simulink model "BANSHEE_SYSTEM"  (Simulink 8.1)
settings: Solver=ode1  StartTime=0.0  StopTime=inf  FixedStep=Ts  MaxStep=1e-3  RelTol=1e-3
model workspace (MAT data in the model file):
  op_snapshot1 : opcond.OperatingPoint (value not decoded)
PostLoadFcn:
  | Ts=100e-6; BANSHEE_init;
InitFcn:
  | Ts=100e-6; BANSHEE_init;
undefined symbols (not defined in the file or in its folder): cable_spec, F1, F2, F3, Feeder1_lib, Feeder2_lib, Feeder3_lib, Left, relay_housing_lib, SM_UtilityService, SS_F1_RELAY_HOUSING, SS_F2_RELAY_HOUSING, SS_F3_RELAY_HOUSING, SS_Feeder1, SS_Feeder2, SS_Feeder3, type, utility_service_lib, V
libraries: breaker_lib x50, relay_modbus_lib x42, rtio_generic_modbus x42, cables_lib x32, artemis x24, transformer_lib x24, Load_lib x18, ssn_lib x16, rtlab x11, powerlib_extras x3, powerlib x2, LoadProfiles_lib x1
(part 1 of 3)
settings Model: ARTEMISmethode_block_infos=$$__separator__$$BANSHEE_SYSTEM/ARTEMIS Guide$$__separator__$$  Creator=RE25624  LastModifiedBy=re25624  BufferReuse=off
settings SolverCC: ZeroCrossAlgorithm=Adaptive
settings DataIOCC: ExternalInput=getinputstruct(op_snapshot1)  InitialState=getstatestruct(op_snapshot1)  LimitDataPoints=off  MaxDataPoints=90060  SignalLoggingSaveFormat=Dataset  SaveOutput=off  SignalLogging=off  DSMLogging=off  SaveTime=off  OutputSaveName=result
settings OptimizationCC: BlockReduction=off  OptimizeBlockIOStorage=off  BufferReuse=off  ExpressionFolding=off  LocalBlockOutputs=off
settings DebuggingCC: MaxConsecutiveZCsMsg=warning  IgnoredZcDiagnostic=none  SolverPrmCheckMsg=none  MultiTaskRateTransMsg=warning  FcnCallInpInsideContextMsg=EnableAllAsWarning  FrameProcessingCompatibilityMsg=error  ModelReferenceExtraNoncontSigs=warning  StrictBusMsg=None
settings ModelReferenceCC: UpdateModelReferenceTargets=IfOutOfDate
settings SFSimCC: SFSimEcho=off
settings GRTTargetCC: CodeReplacementLibrary=C89/C90 (ANSI)

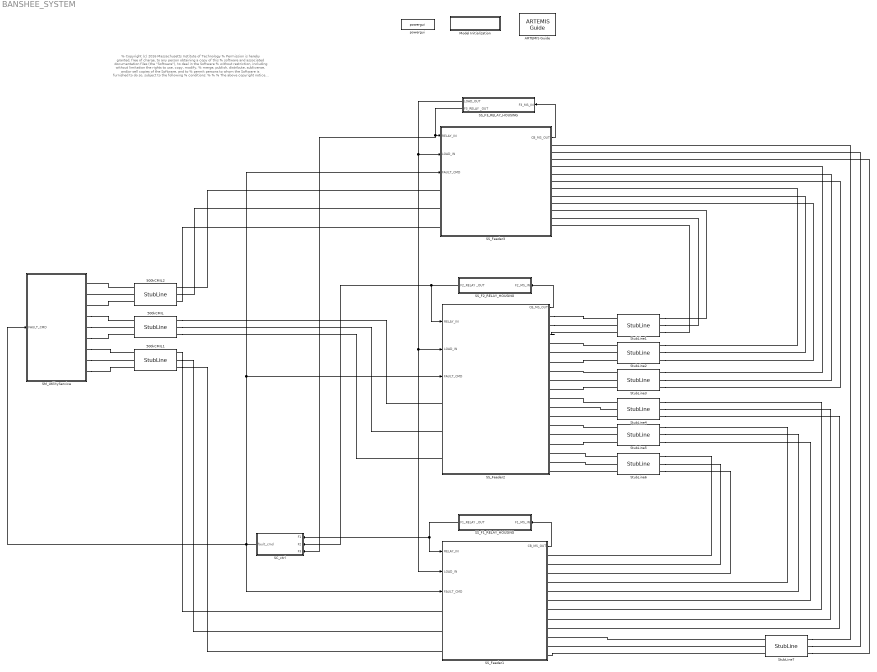
== system BANSHEE_SYSTEM ==
  note: % Copyright (c) 2016 Massachusetts Institute of Technology
      | % Permission is hereby granted, free of charge, to any person obtaining a copy of this
      | % software and associated documentation files (the "Software"), to deal in the Software
      | % without restriction, including without limitation the rights to use, copy, modify,
      | % merge, publish, distribute, sublicense, and/or sell copies of the Software, and to
      | % permit persons to whom the Software is furnished to do so, subject to the following
      | % conditions:
      | %
      | %
      | % The above copyright notice and this permission notice shall be included in
      | % all copies or substantial portions of the Software.
      | %
      | % THE SOFTWARE IS PROVIDED "AS IS", WITHOUT WARRANTY OF ANY KIND, EXPRESS OR IMPLIED,
      | % INCLUDING BUT NOT LIMITED TO THE WARRANTIES OF MERCHANTABILITY, FITNESS FOR A
      | % PARTICULAR PURPOSE AND NONINFRINGEMENT. IN NO EVENT SHALL THE AUTHORS OR COPYRIGHT
      | % HOLDERS BE LIABLE FOR ANY CLAIM, DAMAGES OR OTHER LIABILITY, WHETHER IN AN ACTION
      | % OF CONTRACT, TORT OR OTHERWISE, ARISING FROM, OUT OF OR IN CONNECTION WITH THE
      | % SOFTWARE OR THE USE OR OTHER DEALINGS IN THE SOFTWARE.
      | %
      | %
      | %%
  500kCMIL : artemis/ARTEMIS/StubLine  Phases=3  pu=off  L=10000 * 9.43453e-08 / 1  Lpu=0.08  R=10000 * 2.28409e-5 / 1  Rpu=0.002  S_base=450e6/3  V_base=230e3/sqrt(3)  F_base=60  Ts=Ts
  500kCMIL1 : artemis/ARTEMIS/StubLine  Phases=3  pu=off  L=10000 * 9.43453e-08 / 1  Lpu=0.08  R=10000 * 2.28409e-5 / 1  Rpu=0.002  S_base=450e6/3  V_base=230e3/sqrt(3)  F_base=60  Ts=Ts
  500kCMIL2 : artemis/ARTEMIS/StubLine  Phases=3  pu=off  L=10000 * 9.43453e-08 / 1  Lpu=0.08  R=10000 * 2.28409e-5 / 1  Rpu=0.002  S_base=450e6/3  V_base=230e3/sqrt(3)  F_base=60  Ts=Ts
  ARTEMIS Guide : artemis/ARTEMIS/ARTEMIS Guide  Tag=FTSSmethode_opal_4hx0r99  Description=5.0_z1  lock=on  Ts=Ts  opt=art5  dyna=off  nb_perm=4  RT_fullcomp=off  ssn=on  ssn_itvc=off  ssn_ivic=off  ssn_ext=off  ssn_solver=Art5 with Backward Euler nodal interface  ssn_impulse=off  ssn_quasimpulse=off  ssn_impulse_loop=5  paraExtinctionThy=off  Thy_Impulse=on  dtc=Off  dtc_opt=normal  ao=on  simtype=off  ct_mac=off  lin_mov=off  lsp=[0.001 2]  spike_skip=Disabled  dtc_extra=1  dtc_sws=normal  dtc_pied=0.5  SPSRulesBlock=SPSRules  tre=on  ctmm=off  LF=off  dpl_type=ARTEMiS DPL  rlc_type=off  custom_type=off  para=on  ssn_ImpulseLoopBlockedStateUpdate=5  ssn_mov_iter_number=5  ssn_switch_iter_number=5
  Model Initialization : Subsystem  AncestorBlock=artemis/Tools /Misc/Model Initialization  mask(Model Functions){InitFcnX=Ts=100e-6; BANSHEE_init;, prel=off, posl=on, inif=on, strf=off}
      mask prompts: InitFcnX "Initialisation"; prel "Preload Function"; posl "PostLoad Function"; inif "InitFcn"; strf "StartFcn"
      mask init:
      | currentBlock = gcb;
      | root = bdroot(currentBlock);
      | 
      | if ~strcmp(get_param(root,'BlockDiagramType'),'library')
      |     if prel==1
      |         set_param(root, 'PreLoadFcn', InitFcnX);
      |     else
      |         set_param(root, 'PreLoadFcn', '');
      |     end
      |     if inif==1
      |         set_param(root, 'InitFcn', InitFcnX);
      |     else
      |         set_param(root, 'InitFcn', '');
      |     end
      |     if strf==1
      |         set_param(root, 'StartFcn', InitFcnX);
      |     else
      |         set_param(root, 'StartFcn', '');
      |     end
      |     if posl==1
      |         set_param(root, 'PostLoadFcn', InitFcnX);
      |     else
      |         set_param(root, 'PostLoadFcn', '');
      |     end
      | end
      | 
      | pos = get_param(currentBlock, 'Position');
      | width = pos(3) - pos(1); height = pos(4) - pos(2);
      | txt = [ upper(root) '\n' '- InitFcn. . . . . '  get_param(root, 'InitFcn') ];
      settings: CopyFcn=set_param(gcb,'LinkStatus','inactive')
      mask Display: text(5, height*0.5, txt, 'horizontalAlignment', 'left', 'verticalAlignment', 'middle') ;
  SC_ctrl : Subsystem
  SM_UtilityService : Subsystem  AncestorBlock=utility_service_lib/SM_UtilityService
  SS_F1_RELAY_HOUSING : Subsystem  AncestorBlock=relay_housing_lib/SS_F1_RELAY_HOUSING
  SS_F2_RELAY_HOUSING : Subsystem  AncestorBlock=relay_housing_lib/SS_F2_RELAY_HOUSING
  SS_F3_RELAY_HOUSING : Subsystem  AncestorBlock=relay_housing_lib/SS_F3_RELAY_HOUSING
  SS_Feeder1 : Subsystem  AncestorBlock=Feeder1_lib/SS_Feeder1
  SS_Feeder2 : Subsystem  AncestorBlock=Feeder2_lib/SS_Feeder2
  SS_Feeder3 : Subsystem  AncestorBlock=Feeder3_lib/SS_Feeder3
  StubLine1 : artemis/ARTEMIS/StubLine  Phases=3  pu=off  L=1500 * 9.43453e-08 / 2  Lpu=0.08  R=1500 * 2.28409e-5 / 2  Rpu=0.002  S_base=450e6/3  V_base=230e3/sqrt(3)  F_base=60  Ts=Ts
  StubLine2 : artemis/ARTEMIS/StubLine  Phases=3  pu=off  L=1500 * 9.43453e-08 / 2  Lpu=0.08  R=1500 * 2.28409e-5 / 2  Rpu=0.002  S_base=450e6/3  V_base=230e3/sqrt(3)  F_base=60  Ts=Ts
  StubLine3 : artemis/ARTEMIS/StubLine  Phases=3  pu=off  L=1500 * 9.43453e-08 / 2  Lpu=0.08  R=1500 * 2.28409e-5 / 2  Rpu=0.002  S_base=450e6/3  V_base=230e3/sqrt(3)  F_base=60  Ts=Ts
  StubLine4 : artemis/ARTEMIS/StubLine  Phases=3  pu=off  L=1000 * 9.43453e-08 / 2  Lpu=0.08  R=1000 * 2.28409e-5 / 2  Rpu=0.002  S_base=450e6/3  V_base=230e3/sqrt(3)  F_base=60  Ts=Ts
  StubLine5 : artemis/ARTEMIS/StubLine  Phases=3  pu=off  L=2000 * 9.43453e-08 / 2  Lpu=0.08  R=2000 * 2.28409e-5 / 2  Rpu=0.002  S_base=450e6/3  V_base=230e3/sqrt(3)  F_base=60  Ts=Ts
  StubLine6 : artemis/ARTEMIS/StubLine  Phases=3  pu=off  L=3000 * 9.43453e-08 / 1  Lpu=0.08  R=3000 * 2.28409e-5 / 1  Rpu=0.002  S_base=450e6/3  V_base=230e3/sqrt(3)  F_base=60  Ts=Ts
  StubLine7 : artemis/ARTEMIS/StubLine  Phases=3  pu=off  L=2000 * 9.43453e-08 / 2  Lpu=0.08  R=2000 * 2.28409e-5 / 2  Rpu=0.002  S_base=450e6/3  V_base=230e3/sqrt(3)  F_base=60  Ts=Ts
  powergui : powerlib/powergui  Priority=2  SimulationMode=Discrete  SolverType=Tustin  SampleTime=Ts  frequency=60  SPID=off  DisableSnubberDevices=off  DisableRonSwitches=off  DisableVfSwitches=off  SwTol=0  Interpol=off  DisplayEquations=off  frequencyindice=0  Pbase=100e6  ErrMax=1e-4  Iterations=50  UnitsV=kV  UnitsW=MW  FunctionMessages=off  echomessages=off  HookPort=off  EnableUseOfTLC=off  x0status=blocks  RestoreLinks=warning  ResistiveCurrentMeasurement=off  Frange=logspace(0,3,50)  Ylog=off  Xlog=off  ShowGrid=off  save=off  variable=ZData  structure=0  ZoomFFT=on  StartTime=0.0  cycles=2  DisplayStyle=off  fundamental=60  FreqAxis=off  MaxFrequency=1000  frequencyindicesteady=1  RmsSteady=1  display=off  Ts=0  methode=off
  wires:
  SS_Feeder3/1(CB_MS_OUT) -> SS_F3_RELAY_HOUSING/1(F3_MS_IN)
  SS_F3_RELAY_HOUSING/2(F3_RELAY _OUT) -> SC_ctrl/3(F3), SS_Feeder3/1(RELAY_IN)
  SS_Feeder2/1(CB_MS_OUT) -> SS_F2_RELAY_HOUSING/1(F2_MS_IN)
  SS_F2_RELAY_HOUSING/1(F2_RELAY _OUT) -> SS_Feeder2/1(RELAY_IN), SC_ctrl/2(F2)
  SS_Feeder1/1(CB_MS_OUT) -> SS_F1_RELAY_HOUSING/1(F1_MS_IN)
  SS_F1_RELAY_HOUSING/1(F1_RELAY _OUT) -> SS_Feeder1/1(RELAY_IN), SC_ctrl/1(F1)
  SS_F3_RELAY_HOUSING/1(LOAD_OUT) -> SS_Feeder1/2(LOAD_IN), SS_Feeder2/2(LOAD_IN), SS_Feeder3/2(LOAD_IN)
  SC_ctrl/1(fault_cmd) -> SS_Feeder1/3(FAULT_CMD), SM_UtilityService/1(FAULT_CMD), SS_Feeder3/3(FAULT_CMD), SS_Feeder2/3(FAULT_CMD)
  connections:
  SS_Feeder2/RConn2 -- StubLine1/LConn2
  SS_Feeder2/RConn1 -- StubLine1/LConn1
  SS_Feeder2/RConn3 -- StubLine1/LConn3
  StubLine2/LConn2 -- SS_Feeder2/RConn5
  StubLine2/LConn3 -- SS_Feeder2/RConn6
  StubLine2/LConn1 -- SS_Feeder2/RConn4
  StubLine3/LConn2 -- SS_Feeder2/RConn8
  StubLine3/LConn1 -- SS_Feeder2/RConn7
  StubLine3/LConn3 -- SS_Feeder2/RConn9
  StubLine4/LConn3 -- SS_Feeder2/RConn12
  StubLine4/LConn2 -- SS_Feeder2/RConn11
  StubLine4/LConn1 -- SS_Feeder2/RConn10
  StubLine7/LConn3 -- SS_Feeder1/RConn12
  StubLine7/LConn2 -- SS_Feeder1/RConn11
  StubLine7/LConn1 -- SS_Feeder1/RConn10
  StubLine5/LConn2 -- SS_Feeder2/RConn14
  StubLine5/LConn1 -- SS_Feeder2/RConn13
  StubLine5/LConn3 -- SS_Feeder2/RConn15
  StubLine6/LConn3 -- SS_Feeder2/RConn18
  StubLine6/LConn2 -- SS_Feeder2/RConn17
  StubLine6/LConn1 -- SS_Feeder2/RConn16
  StubLine6/RConn1 -- SS_Feeder1/RConn1
  StubLine6/RConn2 -- SS_Feeder1/RConn2
  StubLine6/RConn3 -- SS_Feeder1/RConn3
  StubLine5/RConn1 -- SS_Feeder1/RConn4
  StubLine5/RConn2 -- SS_Feeder1/RConn5
  StubLine5/RConn3 -- SS_Feeder1/RConn6
  StubLine4/RConn1 -- SS_Feeder1/RConn7
  StubLine4/RConn2 -- SS_Feeder1/RConn8
  StubLine4/RConn3 -- SS_Feeder1/RConn9
  StubLine3/RConn3 -- SS_Feeder3/RConn6
  StubLine3/RConn2 -- SS_Feeder3/RConn5
  StubLine3/RConn1 -- SS_Feeder3/RConn4
  StubLine2/RConn3 -- SS_Feeder3/RConn9
  StubLine2/RConn2 -- SS_Feeder3/RConn8
  StubLine2/RConn1 -- SS_Feeder3/RConn7
  StubLine1/RConn3 -- SS_Feeder3/RConn12
  StubLine1/RConn2 -- SS_Feeder3/RConn11
  StubLine1/RConn1 -- SS_Feeder3/RConn10
  StubLine7/RConn1 -- SS_Feeder3/RConn1
  StubLine7/RConn2 -- SS_Feeder3/RConn2
  StubLine7/RConn3 -- SS_Feeder3/RConn3
  500kCMIL2/LConn2 -- SM_UtilityService/RConn2
  500kCMIL2/LConn1 -- SM_UtilityService/RConn1
  500kCMIL2/LConn3 -- SM_UtilityService/RConn3
  SM_UtilityService/RConn5 -- 500kCMIL/LConn2
  SM_UtilityService/RConn6 -- 500kCMIL/LConn3
  SM_UtilityService/RConn4 -- 500kCMIL/LConn1
  SM_UtilityService/RConn8 -- 500kCMIL1/LConn2
  SM_UtilityService/RConn7 -- 500kCMIL1/LConn1
  SM_UtilityService/RConn9 -- 500kCMIL1/LConn3
  500kCMIL2/RConn3 -- SS_Feeder3/LConn3
  500kCMIL2/RConn2 -- SS_Feeder3/LConn2
  500kCMIL2/RConn1 -- SS_Feeder3/LConn1
  500kCMIL/RConn1 -- SS_Feeder2/LConn1
  500kCMIL/RConn2 -- SS_Feeder2/LConn2
  500kCMIL/RConn3 -- SS_Feeder2/LConn3
  500kCMIL1/RConn1 -- SS_Feeder1/LConn1
  500kCMIL1/RConn2 -- SS_Feeder1/LConn2
  500kCMIL1/RConn3 -- SS_Feeder1/LConn3

== system BANSHEE_SYSTEM/Model Initialization ==

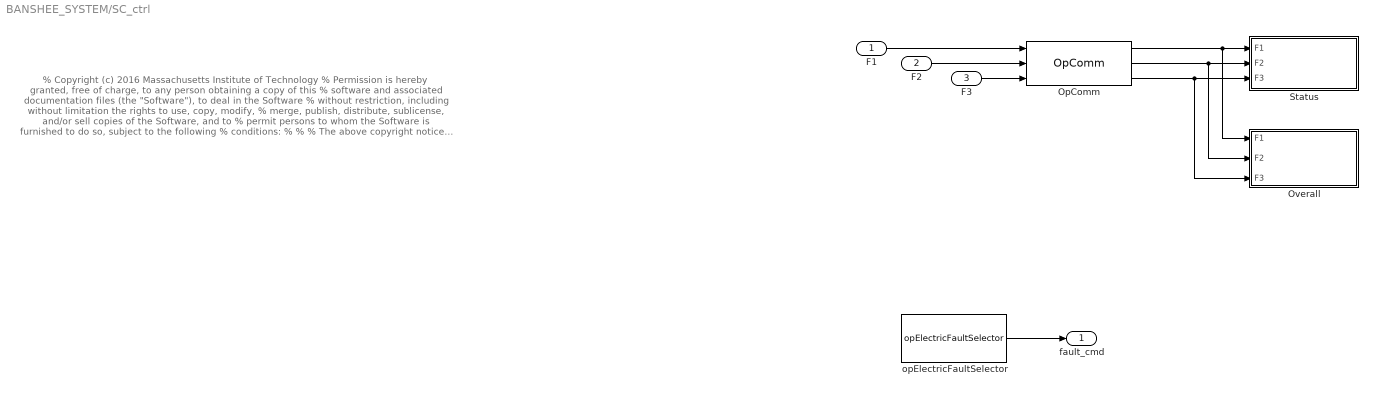
== system BANSHEE_SYSTEM/SC_ctrl ==
  note: % Copyright (c) 2016 Massachusetts Institute of Technology
      | % Permission is hereby granted, free of charge, to any person obtaining a copy of this
      | % software and associated documentation files (the "Software"), to deal in the Software
      | % without restriction, including without limitation the rights to use, copy, modify,
      | % merge, publish, distribute, sublicense, and/or sell copies of the Software, and to
      | % permit persons to whom the Software is furnished to do so, subject to the following
      | % conditions:
      | %
      | %
      | % The above copyright notice and this permission notice shall be included in
      | % all copies or substantial portions of the Software.
      | %
      | % THE SOFTWARE IS PROVIDED "AS IS", WITHOUT WARRANTY OF ANY KIND, EXPRESS OR IMPLIED,
      | % INCLUDING BUT NOT LIMITED TO THE WARRANTIES OF MERCHANTABILITY, FITNESS FOR A
      | % PARTICULAR PURPOSE AND NONINFRINGEMENT. IN NO EVENT SHALL THE AUTHORS OR COPYRIGHT
      | % HOLDERS BE LIABLE FOR ANY CLAIM, DAMAGES OR OTHER LIABILITY, WHETHER IN AN ACTION
      | % OF CONTRACT, TORT OR OTHERWISE, ARISING FROM, OUT OF OR IN CONNECTION WITH THE
      | % SOFTWARE OR THE USE OR OTHER DEALINGS IN THE SOFTWARE.
      | %
      | %
      | %%
  F1 : Inport
  F2 : Inport  Port=2
  F3 : Inport  Port=3
  OpComm : rtlab/OpComm  nbport=3  groupe_acq=1  subsys_rate=0  st=0  Synchronization=on  Interpolation=on  Threshold=1.0  Missed_Data=off  Sim_Time=off  Samples=off  dynSigOut=off  from_console=0  warning_done=off  writeOpCommFile=off  Offset=off
  Overall : Subsystem
  Status : Subsystem
  opElectricFaultSelector : artemis/Tools /POW faults/opElectricFaultSelector  phase_a=on  phase_b=on  phase_c=on  gnd_fault=on  Tacq=1  Tst=[0.1 0 10]  enable_POW=off  angle_POW=[15 0 10]  Tdr="[0.5 0  10]"  fault_location_menu=No fault  T_init=2
  fault_cmd : Outport
  wires:
  F1/1 -> OpComm/1
  F2/1 -> OpComm/2
  F3/1 -> OpComm/3
  OpComm/1 -> Overall/1(F1), Status/1(F1)
  OpComm/2 -> Overall/2(F2), Status/2(F2)
  OpComm/3 -> Overall/3(F3), Status/3(F3)
  opElectricFaultSelector/1 -> fault_cmd/1

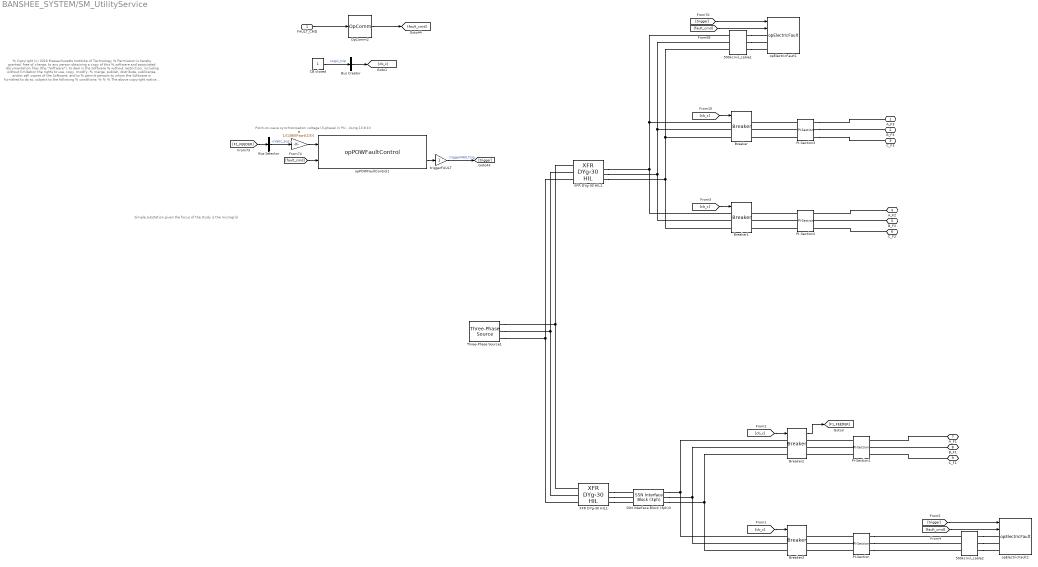
== system BANSHEE_SYSTEM/SM_UtilityService ==
  note: Simple substation given the focus of the study is the microgrid
  note: % Copyright (c) 2016 Massachusetts Institute of Technology
      | % Permission is hereby granted, free of charge, to any person obtaining a copy of this
      | % software and associated documentation files (the "Software"), to deal in the Software
      | % without restriction, including without limitation the rights to use, copy, modify,
      | % merge, publish, distribute, sublicense, and/or sell copies of the Software, and to
      | % permit persons to whom the Software is furnished to do so, subject to the following
      | % conditions:
      | %
      | %
      | % The above copyright notice and this permission notice shall be included in
      | % all copies or substantial portions of the Software.
      | %
      | % THE SOFTWARE IS PROVIDED "AS IS", WITHOUT WARRANTY OF ANY KIND, EXPRESS OR IMPLIED,
      | % INCLUDING BUT NOT LIMITED TO THE WARRANTIES OF MERCHANTABILITY, FITNESS FOR A
      | % PARTICULAR PURPOSE AND NONINFRINGEMENT. IN NO EVENT SHALL THE AUTHORS OR COPYRIGHT
      | % HOLDERS BE LIABLE FOR ANY CLAIM, DAMAGES OR OTHER LIABILITY, WHETHER IN AN ACTION
      | % OF CONTRACT, TORT OR OTHERWISE, ARISING FROM, OUT OF OR IN CONNECTION WITH THE
      | % SOFTWARE OR THE USE OR OTHER DEALINGS IN THE SOFTWARE.
      | %
      | %
      | %%
  note: Point-on-wave synchronisation voltage (3-phase) in PU - Using 13.8 kV
  FAULT_CMD : Inport
  500kcmil_cable1 : cables_lib/500kcmil_cable  length=1  par_sets=1
  500kcmil_cable2 : cables_lib/500kcmil_cable  length=1  par_sets=1
  Breaker{,1..3} (4 alike) : breaker_lib/Breaker  Ts=Ts
  Bus Creator : BusCreator  Inputs=1
  Bus Selector : BusSelector  OutputSignals=Vabc_bus
  CB closed : Constant
  OpComm2 : rtlab/OpComm  nbport=1  groupe_acq=1  subsys_rate=0  st=0  Synchronization=on  Interpolation=on  Threshold=1.0  Missed_Data=off  Sim_Time=off  Samples=off  dynSigOut=off  from_console=1  warning_done=off  writeOpCommFile=off  Offset=off
  PI-Section : cables_lib/PI-Section  cable_spec=[cable_spec(13, :)]  line_length=3000  parallel_sets=1
  PI-Section1 : cables_lib/PI-Section  cable_spec=[cable_spec(13, :)]  line_length=500  parallel_sets=1
  PI-Section2 : cables_lib/PI-Section  cable_spec=[cable_spec(13, :)]  line_length=500  parallel_sets=1
  PI-Section3 : cables_lib/PI-Section  cable_spec=[cable_spec(13, :)]  line_length=500  parallel_sets=1
  SSN Interface Block (3ph)3 : ssn_lib/SSN Interface Block (3ph)  nb_phase=3  nb_port=2  p1_type=V-type(Left)  p2_type=V-type (Right)  p3_type=V-type(Left)  p4_type=V-type(Left)  p5_type=V-type(Left)  p6_type=V-type(Left)  p7_type=V-type(Left)  p8_type=V-type(Left)  p9_type=V-type(Left)  p10_type=V-type(Left)  p11_type=V-type(Left)  p12_type=V-type(Left)  p13_type=V-type(Left)  p14_type=V-type(Left)  p15_type=V-type(Left)  p16_type=V-type(Left)  I_port_shunt_resistance=1e9
  Three-Phase Source1 : powerlib/Electrical Sources/Three-Phase Source  Voltage=115000  PhaseAngle=0  Frequency=60  InternalConnection=Yg  SpecifyImpedance=on  Resistance=0.8929  Inductance=16.58e-3  ShortCircuitLevel=100e6  BaseVoltage=115000  XRratio=30  BusType=swing  Pref=0  Qref=0  Qmin=-inf  Qmax=inf
  XFR DYg-30 HIL1 : transformer_lib/XFR DYg-30 HIL  Rating=50000  Vp=115000  Vs=13800  Z=15  XR=30
  XFR DYg-30 HIL2 : transformer_lib/XFR DYg-30 HIL  Rating=50000  Vp=115000  Vs=13800  Z=15  XR=30
  a : Gain  Gain=1/(13800*sqrt(2/3))
  opElectricFault1 : artemis/Tools /POW faults/opElectricFault  FaultLocation=location 7  FaultResistance=0.0001  GroundResistance=0.0001  InitialStates=[0 0 0]  SnubberResistance=1e6  SnubberCapacitance=inf
  opElectricFault2 : artemis/Tools /POW faults/opElectricFault  FaultLocation=location 8  FaultResistance=0.0001  GroundResistance=0.0001  InitialStates=[0 0 0]  SnubberResistance=1e6  SnubberCapacitance=inf
  opPOWFaultControl1 : artemis/Tools /POW faults/opPOWFaultControl  Ts=Ts  usePLL=off  Fgrid=60  PLL_k=[180 3200 1]  vol_sel=1: rising zero-corssing  SyncPhase_menu=A  T_acq=0.8
  triggerFAULT : Gain
  A_F3 : PMIOPort  Port=1  Side=Right
  B_F3 : PMIOPort  Port=2  Side=Right
  C_F3 : PMIOPort  Port=3  Side=Right
  A_F2 : PMIOPort  Port=4  Side=Right
  B_F2 : PMIOPort  Port=5  Side=Right
  C_F2 : PMIOPort  Port=6  Side=Right
  A_F1 : PMIOPort  Port=7  Side=Right
  B_F1 : PMIOPort  Port=8  Side=Right
  C_F1 : PMIOPort  Port=9  Side=Right
  wires:
  [cb_c] -> Breaker2/1
  [cb_c] -> Breaker/1
  [cb_c] -> Breaker1/1
  [cb_c] -> Breaker3/1
  Bus Creator/1 -> [cb_c]
  CB closed/1 -> Bus Creator/1  "Logic_trip"
  [fault_cmd] -> opElectricFault1/2
  [trigger] -> opElectricFault1/1
  [fault_cmd] -> opPOWFaultControl1/2
  opPOWFaultControl1/2 -> triggerFAULT/1
  triggerFAULT/1 -> [trigger]  "triggerFAULTsig"
  [F1_FEEDER] -> Bus Selector/1
  Bus Selector/1 -> a/1  "<Vabc_bus>"
  a/1 -> opPOWFaultControl1/1
  OpComm2/1 -> [fault_cmd]
  FAULT_CMD/1 -> OpComm2/1
  Breaker2/1 -> [F1_FEEDER]
  [fault_cmd] -> opElectricFault2/2
  [trigger] -> opElectricFault2/1
  connections:
  PI-Section2/LConn1 -- Breaker1/RConn1
  PI-Section2/LConn3 -- Breaker1/RConn3
  PI-Section1/LConn1 -- Breaker2/RConn1
  PI-Section1/LConn2 -- Breaker2/RConn2
  PI-Section3/LConn1 -- Breaker/RConn1
  PI-Section1/LConn3 -- Breaker2/RConn3
  Breaker3/LConn2 -- SSN Interface Block (3ph)3/RConn2 -- Breaker2/LConn2
  PI-Section3/LConn2 -- Breaker/RConn2
  Breaker3/LConn3 -- SSN Interface Block (3ph)3/RConn3 -- Breaker2/LConn3
  PI-Section/LConn3 -- Breaker3/RConn3
  PI-Section2/LConn2 -- Breaker1/RConn2
  PI-Section/LConn1 -- Breaker3/RConn1
  Breaker3/LConn1 -- SSN Interface Block (3ph)3/RConn1 -- Breaker2/LConn1
  PI-Section3/LConn3 -- Breaker/RConn3
  Breaker1/LConn2 -- 500kcmil_cable1/LConn2 -- Breaker/LConn2 -- XFR DYg-30 HIL2/RConn2
  XFR DYg-30 HIL2/RConn1 -- Breaker1/LConn1 -- 500kcmil_cable1/LConn1 -- Breaker/LConn1
  Breaker1/LConn3 -- 500kcmil_cable1/LConn3 -- Breaker/LConn3 -- XFR DYg-30 HIL2/RConn3
  PI-Section/LConn2 -- Breaker3/RConn2
  A_F2/RConn1 -- PI-Section2/RConn1
  B_F1/RConn1 -- PI-Section1/RConn2
  PI-Section3/RConn3 -- C_F3/RConn1
  Three-Phase Source1/RConn3 -- XFR DYg-30 HIL2/LConn3 -- XFR DYg-30 HIL1/LConn3
  Three-Phase Source1/RConn2 -- XFR DYg-30 HIL2/LConn2 -- XFR DYg-30 HIL1/LConn2
  Three-Phase Source1/RConn1 -- XFR DYg-30 HIL2/LConn1 -- XFR DYg-30 HIL1/LConn1
  C_F2/RConn1 -- PI-Section2/RConn3
  PI-Section3/RConn1 -- A_F3/RConn1
  B_F2/RConn1 -- PI-Section2/RConn2
  A_F1/RConn1 -- PI-Section1/RConn1
  C_F1/RConn1 -- PI-Section1/RConn3
  PI-Section3/RConn2 -- B_F3/RConn1
  500kcmil_cable1/RConn3 -- opElectricFault1/LConn3
  500kcmil_cable1/RConn2 -- opElectricFault1/LConn2
  500kcmil_cable1/RConn1 -- opElectricFault1/LConn1
  500kcmil_cable2/RConn3 -- opElectricFault2/LConn3
  500kcmil_cable2/RConn2 -- opElectricFault2/LConn2
  500kcmil_cable2/RConn1 -- opElectricFault2/LConn1
  PI-Section/RConn3 -- 500kcmil_cable2/LConn3
  PI-Section/RConn2 -- 500kcmil_cable2/LConn2
  PI-Section/RConn1 -- 500kcmil_cable2/LConn1
  XFR DYg-30 HIL1/RConn3 -- SSN Interface Block (3ph)3/LConn3
  XFR DYg-30 HIL1/RConn2 -- SSN Interface Block (3ph)3/LConn2
  XFR DYg-30 HIL1/RConn1 -- SSN Interface Block (3ph)3/LConn1

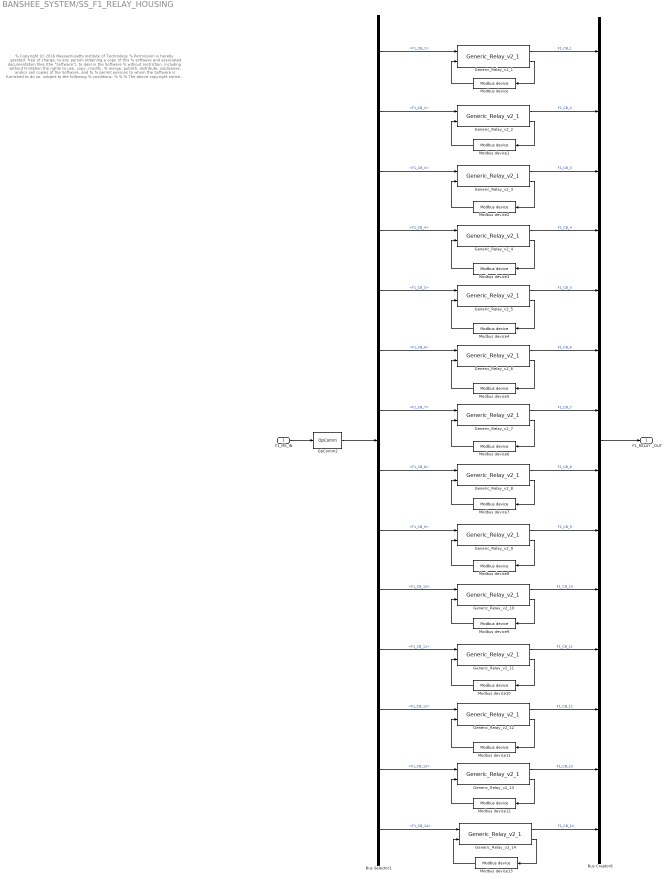
== system BANSHEE_SYSTEM/SS_F1_RELAY_HOUSING ==
  note: % Copyright (c) 2016 Massachusetts Institute of Technology
      | % Permission is hereby granted, free of charge, to any person obtaining a copy of this
      | % software and associated documentation files (the "Software"), to deal in the Software
      | % without restriction, including without limitation the rights to use, copy, modify,
      | % merge, publish, distribute, sublicense, and/or sell copies of the Software, and to
      | % permit persons to whom the Software is furnished to do so, subject to the following
      | % conditions:
      | %
      | %
      | % The above copyright notice and this permission notice shall be included in
      | % all copies or substantial portions of the Software.
      | %
      | % THE SOFTWARE IS PROVIDED "AS IS", WITHOUT WARRANTY OF ANY KIND, EXPRESS OR IMPLIED,
      | % INCLUDING BUT NOT LIMITED TO THE WARRANTIES OF MERCHANTABILITY, FITNESS FOR A
      | % PARTICULAR PURPOSE AND NONINFRINGEMENT. IN NO EVENT SHALL THE AUTHORS OR COPYRIGHT
      | % HOLDERS BE LIABLE FOR ANY CLAIM, DAMAGES OR OTHER LIABILITY, WHETHER IN AN ACTION
      | % OF CONTRACT, TORT OR OTHERWISE, ARISING FROM, OUT OF OR IN CONNECTION WITH THE
      | % SOFTWARE OR THE USE OR OTHER DEALINGS IN THE SOFTWARE.
      | %
      | %
      | %%
  F1_MS_IN : Inport
  Bus Creator6 : BusCreator  Inputs=14
  Bus Selector1 : BusSelector  OutputSignals=F1_CB_1,F1_CB_2,F1_CB_3,F1_CB_4,F1_CB_5,F1_CB_6,F1_CB_7,F1_CB_8,F1_CB_9,F1_CB_10,F1_CB_11,F1_CB_12,F1_CB_13,F1_CB_14
  Generic_Relay_v2_1 : relay_modbus_lib/Generic_Relay_v2_1  Ts=Ts  relay_settings=[F1(1,:)]
  Generic_Relay_v2_10 : relay_modbus_lib/Generic_Relay_v2_1  Ts=Ts  relay_settings=[F1(10,:)]
  Generic_Relay_v2_11 : relay_modbus_lib/Generic_Relay_v2_1  Ts=Ts  relay_settings=[F1(11,:)]
  Generic_Relay_v2_12 : relay_modbus_lib/Generic_Relay_v2_1  Ts=Ts  relay_settings=[F1(12,:)]
  Generic_Relay_v2_13 : relay_modbus_lib/Generic_Relay_v2_1  Ts=Ts  relay_settings=[F1(13,:)]
  Generic_Relay_v2_14 : relay_modbus_lib/Generic_Relay_v2_1  Ts=Ts  relay_settings=[F1(14,:)]
  Generic_Relay_v2_2 : relay_modbus_lib/Generic_Relay_v2_1  Ts=Ts  relay_settings=[F1(2,:)]
  Generic_Relay_v2_3 : relay_modbus_lib/Generic_Relay_v2_1  Ts=Ts  relay_settings=[F1(3,:)]
  Generic_Relay_v2_4 : relay_modbus_lib/Generic_Relay_v2_1  Ts=Ts  relay_settings=[F1(4,:)]
  Generic_Relay_v2_5 : relay_modbus_lib/Generic_Relay_v2_1  Ts=Ts  relay_settings=[F1(5,:)]
  Generic_Relay_v2_6 : relay_modbus_lib/Generic_Relay_v2_1  Ts=Ts  relay_settings=[F1(6,:)]
  Generic_Relay_v2_7 : relay_modbus_lib/Generic_Relay_v2_1  Ts=Ts  relay_settings=[F1(7,:)]
  Generic_Relay_v2_8 : relay_modbus_lib/Generic_Relay_v2_1  Ts=Ts  relay_settings=[F1(8,:)]
  Generic_Relay_v2_9 : relay_modbus_lib/Generic_Relay_v2_1  Ts=Ts  relay_settings=[F1(9,:)]
  Modbus device : rtio_generic_modbus/Modbus device  conf_name=F1_relay_cfg1.opal  conf_name_mask=F1_relay_cfg1.xls  sample_time=Ts
  Modbus device1 : rtio_generic_modbus/Modbus device  conf_name=F1_relay_cfg2.opal  conf_name_mask=F1_relay_cfg2.xls  sample_time=Ts
  Modbus device10 : rtio_generic_modbus/Modbus device  conf_name=F1_relay_cfg11.opal  conf_name_mask=F1_relay_cfg11.xls  sample_time=Ts
  Modbus device11 : rtio_generic_modbus/Modbus device  conf_name=F1_relay_cfg12.opal  conf_name_mask=F1_relay_cfg12.xls  sample_time=Ts
  Modbus device12 : rtio_generic_modbus/Modbus device  conf_name=F1_relay_cfg13.opal  conf_name_mask=F1_relay_cfg13.xls  sample_time=Ts
  Modbus device13 : rtio_generic_modbus/Modbus device  conf_name=F1_relay_cfg14.opal  conf_name_mask=F1_relay_cfg14.xls  sample_time=Ts
  Modbus device2 : rtio_generic_modbus/Modbus device  conf_name=F1_relay_cfg3.opal  conf_name_mask=F1_relay_cfg3.xls  sample_time=Ts
  Modbus device3 : rtio_generic_modbus/Modbus device  conf_name=F1_relay_cfg4.opal  conf_name_mask=F1_relay_cfg4.xls  sample_time=Ts
  Modbus device4 : rtio_generic_modbus/Modbus device  conf_name=F1_relay_cfg5.opal  conf_name_mask=F1_relay_cfg5.xls  sample_time=Ts
  Modbus device5 : rtio_generic_modbus/Modbus device  conf_name=F1_relay_cfg6.opal  conf_name_mask=F1_relay_cfg6.xls  sample_time=Ts
  Modbus device6 : rtio_generic_modbus/Modbus device  conf_name=F1_relay_cfg7.opal  conf_name_mask=F1_relay_cfg7.xls  sample_time=Ts
  Modbus device7 : rtio_generic_modbus/Modbus device  conf_name=F1_relay_cfg8.opal  conf_name_mask=F1_relay_cfg8.xls  sample_time=Ts
  Modbus device8 : rtio_generic_modbus/Modbus device  conf_name=F1_relay_cfg9.opal  conf_name_mask=F1_relay_cfg9.xls  sample_time=Ts
  Modbus device9 : rtio_generic_modbus/Modbus device  conf_name=F1_relay_cfg10.opal  conf_name_mask=F1_relay_cfg10.xls  sample_time=Ts
  OpComm2 : rtlab/OpComm  nbport=1  groupe_acq=1  subsys_rate=0  st=0  Synchronization=on  Interpolation=on  Threshold=1.0  Missed_Data=off  Sim_Time=off  Samples=off  dynSigOut=off  from_console=0  warning_done=off  writeOpCommFile=off  Offset=off
  F1_RELAY _OUT : Outport
  wires:
  OpComm2/1 -> Bus Selector1/1
  Modbus device12/1 -> Generic_Relay_v2_13/2
  Generic_Relay_v2_13/2 -> Modbus device12/1
  Modbus device11/1 -> Generic_Relay_v2_12/2
  Generic_Relay_v2_12/2 -> Modbus device11/1
  Modbus device10/1 -> Generic_Relay_v2_11/2
  Generic_Relay_v2_11/2 -> Modbus device10/1
  Modbus device9/1 -> Generic_Relay_v2_10/2
  Generic_Relay_v2_10/2 -> Modbus device9/1
  Modbus device8/1 -> Generic_Relay_v2_9/2
  Generic_Relay_v2_9/2 -> Modbus device8/1
  Modbus device7/1 -> Generic_Relay_v2_8/2
  Generic_Relay_v2_8/2 -> Modbus device7/1
  Modbus device6/1 -> Generic_Relay_v2_7/2
  Generic_Relay_v2_7/2 -> Modbus device6/1
  Modbus device5/1 -> Generic_Relay_v2_6/2
  Generic_Relay_v2_6/2 -> Modbus device5/1
  Modbus device4/1 -> Generic_Relay_v2_5/2
  Generic_Relay_v2_5/2 -> Modbus device4/1
  Modbus device3/1 -> Generic_Relay_v2_4/2
  Generic_Relay_v2_4/2 -> Modbus device3/1
  Modbus device2/1 -> Generic_Relay_v2_3/2
  Generic_Relay_v2_3/2 -> Modbus device2/1
  Generic_Relay_v2_2/2 -> Modbus device1/1
  Modbus device1/1 -> Generic_Relay_v2_2/2
  Generic_Relay_v2_1/2 -> Modbus device/1
  Modbus device/1 -> Generic_Relay_v2_1/2
  F1_MS_IN/1 -> OpComm2/1
  Bus Selector1/1 -> Generic_Relay_v2_1/1  "<F1_CB_1>"
  Generic_Relay_v2_1/1 -> Bus Creator6/1  "F1_CB_1"
  Bus Creator6/1 -> F1_RELAY _OUT/1
  Bus Selector1/2 -> Generic_Relay_v2_2/1  "<F1_CB_2>"
  Generic_Relay_v2_2/1 -> Bus Creator6/2  "F1_CB_2"
  Bus Selector1/3 -> Generic_Relay_v2_3/1  "<F1_CB_3>"
  Bus Selector1/4 -> Generic_Relay_v2_4/1  "<F1_CB_4>"
  Bus Selector1/5 -> Generic_Relay_v2_5/1  "<F1_CB_5>"
  Bus Selector1/6 -> Generic_Relay_v2_6/1  "<F1_CB_6>"
  Bus Selector1/7 -> Generic_Relay_v2_7/1  "<F1_CB_7>"
  Bus Selector1/8 -> Generic_Relay_v2_8/1  "<F1_CB_8>"
  Bus Selector1/9 -> Generic_Relay_v2_9/1  "<F1_CB_9>"
  Bus Selector1/10 -> Generic_Relay_v2_10/1  "<F1_CB_10>"
  Bus Selector1/11 -> Generic_Relay_v2_11/1  "<F1_CB_11>"
  Bus Selector1/12 -> Generic_Relay_v2_12/1  "<F1_CB_12>"
  Bus Selector1/13 -> Generic_Relay_v2_13/1  "<F1_CB_13>"
  Generic_Relay_v2_13/1 -> Bus Creator6/13  "F1_CB_13"
  Generic_Relay_v2_12/1 -> Bus Creator6/12  "F1_CB_12"
  Generic_Relay_v2_11/1 -> Bus Creator6/11  "F1_CB_11"
  Generic_Relay_v2_10/1 -> Bus Creator6/10  "F1_CB_10"
  Generic_Relay_v2_9/1 -> Bus Creator6/9  "F1_CB_9"
  Generic_Relay_v2_8/1 -> Bus Creator6/8  "F1_CB_8"
  Generic_Relay_v2_7/1 -> Bus Creator6/7  "F1_CB_7"
  Generic_Relay_v2_6/1 -> Bus Creator6/6  "F1_CB_6"
  Generic_Relay_v2_5/1 -> Bus Creator6/5  "F1_CB_5"
  Generic_Relay_v2_4/1 -> Bus Creator6/4  "F1_CB_4"
  Generic_Relay_v2_3/1 -> Bus Creator6/3  "F1_CB_3"
  Modbus device13/1 -> Generic_Relay_v2_14/2
  Generic_Relay_v2_14/2 -> Modbus device13/1
  Generic_Relay_v2_14/1 -> Bus Creator6/14  "F1_CB_14"
  Bus Selector1/14 -> Generic_Relay_v2_14/1  "<F1_CB_14>"

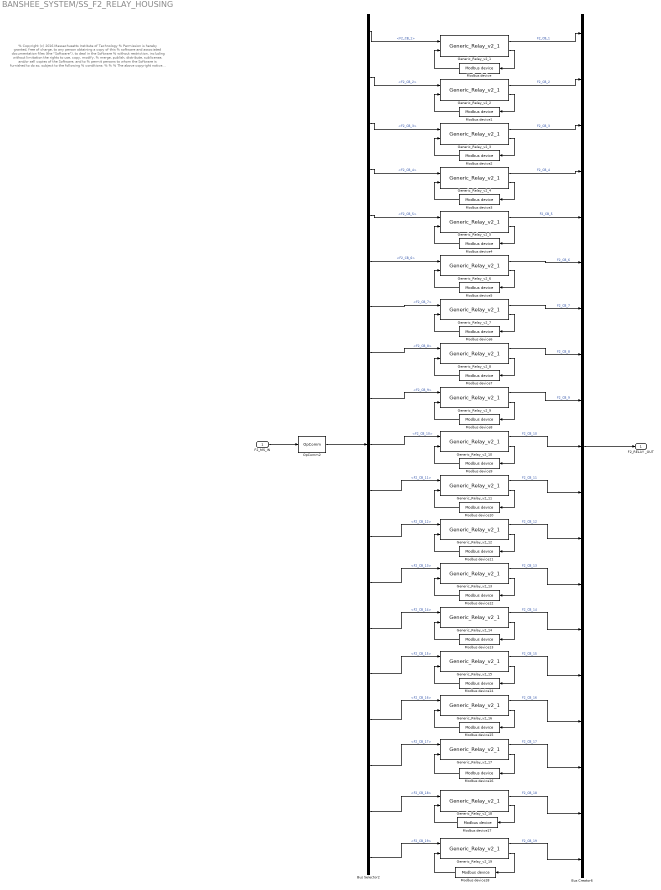
== system BANSHEE_SYSTEM/SS_F2_RELAY_HOUSING ==
  note: % Copyright (c) 2016 Massachusetts Institute of Technology
      | % Permission is hereby granted, free of charge, to any person obtaining a copy of this
      | % software and associated documentation files (the "Software"), to deal in the Software
      | % without restriction, including without limitation the rights to use, copy, modify,
      | % merge, publish, distribute, sublicense, and/or sell copies of the Software, and to
      | % permit persons to whom the Software is furnished to do so, subject to the following
      | % conditions:
      | %
      | %
      | % The above copyright notice and this permission notice shall be included in
      | % all copies or substantial portions of the Software.
      | %
      | % THE SOFTWARE IS PROVIDED "AS IS", WITHOUT WARRANTY OF ANY KIND, EXPRESS OR IMPLIED,
      | % INCLUDING BUT NOT LIMITED TO THE WARRANTIES OF MERCHANTABILITY, FITNESS FOR A
      | % PARTICULAR PURPOSE AND NONINFRINGEMENT. IN NO EVENT SHALL THE AUTHORS OR COPYRIGHT
      | % HOLDERS BE LIABLE FOR ANY CLAIM, DAMAGES OR OTHER LIABILITY, WHETHER IN AN ACTION
      | % OF CONTRACT, TORT OR OTHERWISE, ARISING FROM, OUT OF OR IN CONNECTION WITH THE
      | % SOFTWARE OR THE USE OR OTHER DEALINGS IN THE SOFTWARE.
      | %
      | %
      | %%
  F2_MS_IN : Inport
  Bus Creator6 : BusCreator  Inputs=19
  Bus Selector2 : BusSelector  OutputSignals=F2_CB_1,F2_CB_2,F2_CB_3,F2_CB_4,F2_CB_5,F2_CB_6,F2_CB_7,F2_CB_8,F2_CB_9,F2_CB_10,F2_CB_11,F2_CB_12,F2_CB_13,F2_CB_14,F2_CB_15,F2_CB_16,F2_CB_17,F2_CB_18,F2_CB_19
  Generic_Relay_v2_1 : relay_modbus_lib/Generic_Relay_v2_1  Ts=Ts  relay_settings=[F2(1,:)]
  Generic_Relay_v2_10 : relay_modbus_lib/Generic_Relay_v2_1  Ts=Ts  relay_settings=[F2(10,:)]
  Generic_Relay_v2_11 : relay_modbus_lib/Generic_Relay_v2_1  Ts=Ts  relay_settings=[F2(11,:)]
  Generic_Relay_v2_12 : relay_modbus_lib/Generic_Relay_v2_1  Ts=Ts  relay_settings=[F2(12,:)]
  Generic_Relay_v2_13 : relay_modbus_lib/Generic_Relay_v2_1  Ts=Ts  relay_settings=[F2(13,:)]
  Generic_Relay_v2_14 : relay_modbus_lib/Generic_Relay_v2_1  Ts=Ts  relay_settings=[F2(14,:)]
  Generic_Relay_v2_15 : relay_modbus_lib/Generic_Relay_v2_1  Ts=Ts  relay_settings=[F2(15,:)]
  Generic_Relay_v2_16 : relay_modbus_lib/Generic_Relay_v2_1  Ts=Ts  relay_settings=[F2(16,:)]
  Generic_Relay_v2_17 : relay_modbus_lib/Generic_Relay_v2_1  Ts=Ts  relay_settings=[F2(17,:)]
  Generic_Relay_v2_18 : relay_modbus_lib/Generic_Relay_v2_1  Ts=Ts  relay_settings=[F2(18,:)]
  Generic_Relay_v2_19 : relay_modbus_lib/Generic_Relay_v2_1  Ts=Ts  relay_settings=[F2(19,:)]
  Generic_Relay_v2_2 : relay_modbus_lib/Generic_Relay_v2_1  Ts=Ts  relay_settings=[F2(2,:)]
  Generic_Relay_v2_3 : relay_modbus_lib/Generic_Relay_v2_1  Ts=Ts  relay_settings=[F2(3,:)]
  Generic_Relay_v2_4 : relay_modbus_lib/Generic_Relay_v2_1  Ts=Ts  relay_settings=[F2(4,:)]
  Generic_Relay_v2_5 : relay_modbus_lib/Generic_Relay_v2_1  Ts=Ts  relay_settings=[F2(5,:)]
  Generic_Relay_v2_6 : relay_modbus_lib/Generic_Relay_v2_1  Ts=Ts  relay_settings=[F2(6,:)]
  Generic_Relay_v2_7 : relay_modbus_lib/Generic_Relay_v2_1  Ts=Ts  relay_settings=[F2(7,:)]
  Generic_Relay_v2_8 : relay_modbus_lib/Generic_Relay_v2_1  Ts=Ts  relay_settings=[F2(8,:)]
  Generic_Relay_v2_9 : relay_modbus_lib/Generic_Relay_v2_1  Ts=Ts  relay_settings=[F2(9,:)]
  Modbus device : rtio_generic_modbus/Modbus device  conf_name=F2_relay_cfg1.opal  conf_name_mask=F2_relay_cfg1.xls  sample_time=Ts
  Modbus device1 : rtio_generic_modbus/Modbus device  conf_name=F2_relay_cfg2.opal  conf_name_mask=F2_relay_cfg2.xls  sample_time=Ts
  Modbus device10 : rtio_generic_modbus/Modbus device  conf_name=F2_relay_cfg11.opal  conf_name_mask=F2_relay_cfg11.xls  sample_time=Ts
  Modbus device11 : rtio_generic_modbus/Modbus device  conf_name=F2_relay_cfg12.opal  conf_name_mask=F2_relay_cfg12.xls  sample_time=Ts
  Modbus device12 : rtio_generic_modbus/Modbus device  conf_name=F2_relay_cfg13.opal  conf_name_mask=F2_relay_cfg13.xls  sample_time=Ts
  Modbus device13 : rtio_generic_modbus/Modbus device  conf_name=F2_relay_cfg14.opal  conf_name_mask=F2_relay_cfg14.xls  sample_time=Ts
  Modbus device14 : rtio_generic_modbus/Modbus device  conf_name=F2_relay_cfg15.opal  conf_name_mask=F2_relay_cfg15.xls  sample_time=Ts
  Modbus device15 : rtio_generic_modbus/Modbus device  conf_name=F2_relay_cfg16.opal  conf_name_mask=F2_relay_cfg16.xls  sample_time=Ts
  Modbus device16 : rtio_generic_modbus/Modbus device  conf_name=F2_relay_cfg17.opal  conf_name_mask=F2_relay_cfg17.xls  sample_time=Ts
  Modbus device17 : rtio_generic_modbus/Modbus device  conf_name=F2_relay_cfg18.opal  conf_name_mask=F2_relay_cfg18.xls  sample_time=Ts
  Modbus device18 : rtio_generic_modbus/Modbus device  conf_name=F2_relay_cfg19.opal  conf_name_mask=F2_relay_cfg19.xls  sample_time=Ts
  Modbus device2 : rtio_generic_modbus/Modbus device  conf_name=F2_relay_cfg3.opal  conf_name_mask=F2_relay_cfg3.xls  sample_time=Ts
  Modbus device3 : rtio_generic_modbus/Modbus device  conf_name=F2_relay_cfg4.opal  conf_name_mask=F2_relay_cfg4.xls  sample_time=Ts
  Modbus device4 : rtio_generic_modbus/Modbus device  conf_name=F2_relay_cfg5.opal  conf_name_mask=F2_relay_cfg5.xls  sample_time=Ts
  Modbus device5 : rtio_generic_modbus/Modbus device  conf_name=F2_relay_cfg6.opal  conf_name_mask=F2_relay_cfg6.xls  sample_time=Ts
  Modbus device6 : rtio_generic_modbus/Modbus device  conf_name=F2_relay_cfg7.opal  conf_name_mask=F2_relay_cfg7.xls  sample_time=Ts
  Modbus device7 : rtio_generic_modbus/Modbus device  conf_name=F2_relay_cfg8.opal  conf_name_mask=F2_relay_cfg8.xls  sample_time=Ts
  Modbus device8 : rtio_generic_modbus/Modbus device  conf_name=F2_relay_cfg9.opal  conf_name_mask=F2_relay_cfg9.xls  sample_time=Ts
  Modbus device9 : rtio_generic_modbus/Modbus device  conf_name=F2_relay_cfg10.opal  conf_name_mask=F2_relay_cfg10.xls  sample_time=Ts
  OpComm2 : rtlab/OpComm  nbport=1  groupe_acq=1  subsys_rate=0  st=0  Synchronization=on  Interpolation=on  Threshold=1.0  Missed_Data=off  Sim_Time=off  Samples=off  dynSigOut=off  from_console=0  warning_done=off  writeOpCommFile=off  Offset=off
  F2_RELAY _OUT : Outport
  wires:
  OpComm2/1 -> Bus Selector2/1
  Modbus device16/1 -> Generic_Relay_v2_17/2
  Generic_Relay_v2_17/2 -> Modbus device16/1
  Modbus device15/1 -> Generic_Relay_v2_16/2
  Generic_Relay_v2_16/2 -> Modbus device15/1
  Modbus device14/1 -> Generic_Relay_v2_15/2
  Generic_Relay_v2_15/2 -> Modbus device14/1
  Modbus device13/1 -> Generic_Relay_v2_14/2
  Generic_Relay_v2_14/2 -> Modbus device13/1
  Generic_Relay_v2_13/2 -> Modbus device12/1
  Modbus device12/1 -> Generic_Relay_v2_13/2
  Modbus device11/1 -> Generic_Relay_v2_12/2
  Generic_Relay_v2_12/2 -> Modbus device11/1
  Modbus device10/1 -> Generic_Relay_v2_11/2
  Generic_Relay_v2_11/2 -> Modbus device10/1
  Modbus device9/1 -> Generic_Relay_v2_10/2
  Generic_Relay_v2_10/2 -> Modbus device9/1
  Modbus device8/1 -> Generic_Relay_v2_9/2
  Generic_Relay_v2_9/2 -> Modbus device8/1
  Modbus device7/1 -> Generic_Relay_v2_8/2
  Generic_Relay_v2_8/2 -> Modbus device7/1
  Modbus device6/1 -> Generic_Relay_v2_7/2
  Generic_Relay_v2_7/2 -> Modbus device6/1
  Generic_Relay_v2_6/2 -> Modbus device5/1
  Modbus device5/1 -> Generic_Relay_v2_6/2
  Modbus device4/1 -> Generic_Relay_v2_5/2
  Generic_Relay_v2_5/2 -> Modbus device4/1
  Modbus device3/1 -> Generic_Relay_v2_4/2
  Generic_Relay_v2_4/2 -> Modbus device3/1
  Modbus device2/1 -> Generic_Relay_v2_3/2
  Generic_Relay_v2_3/2 -> Modbus device2/1
  Modbus device1/1 -> Generic_Relay_v2_2/2
  Generic_Relay_v2_2/2 -> Modbus device1/1
  Modbus device/1 -> Generic_Relay_v2_1/2
  Generic_Relay_v2_1/2 -> Modbus device/1
  Bus Creator6/1 -> F2_RELAY _OUT/1
  F2_MS_IN/1 -> OpComm2/1
  Bus Selector2/1 -> Generic_Relay_v2_1/1  "<F2_CB_1>"
  Generic_Relay_v2_1/1 -> Bus Creator6/1  "F2_CB_1"
  Bus Selector2/2 -> Generic_Relay_v2_2/1  "<F2_CB_2>"
  Bus Selector2/3 -> Generic_Relay_v2_3/1  "<F2_CB_3>"
  Bus Selector2/4 -> Generic_Relay_v2_4/1  "<F2_CB_4>"
  Bus Selector2/5 -> Generic_Relay_v2_5/1  "<F2_CB_5>"
  Bus Selector2/6 -> Generic_Relay_v2_6/1  "<F2_CB_6>"
  Bus Selector2/7 -> Generic_Relay_v2_7/1  "<F2_CB_7>"
  Bus Selector2/8 -> Generic_Relay_v2_8/1  "<F2_CB_8>"
  Bus Selector2/9 -> Generic_Relay_v2_9/1  "<F2_CB_9>"
  Bus Selector2/10 -> Generic_Relay_v2_10/1  "<F2_CB_10>"
  Bus Selector2/11 -> Generic_Relay_v2_11/1  "<F2_CB_11>"
  Bus Selector2/12 -> Generic_Relay_v2_12/1  "<F2_CB_12>"
  Bus Selector2/13 -> Generic_Relay_v2_13/1  "<F2_CB_13>"
  Bus Selector2/14 -> Generic_Relay_v2_14/1  "<F2_CB_14>"
  Bus Selector2/15 -> Generic_Relay_v2_15/1  "<F2_CB_15>"
  Bus Selector2/16 -> Generic_Relay_v2_16/1  "<F2_CB_16>"
  Generic_Relay_v2_12/1 -> Bus Creator6/12  "F2_CB_12"
  Generic_Relay_v2_13/1 -> Bus Creator6/13  "F2_CB_13"
  Generic_Relay_v2_14/1 -> Bus Creator6/14  "F2_CB_14"
  Generic_Relay_v2_15/1 -> Bus Creator6/15  "F2_CB_15"
  Generic_Relay_v2_16/1 -> Bus Creator6/16  "F2_CB_16"
  Generic_Relay_v2_11/1 -> Bus Creator6/11  "F2_CB_11"
  Generic_Relay_v2_10/1 -> Bus Creator6/10  "F2_CB_10"
  Generic_Relay_v2_9/1 -> Bus Creator6/9  "F2_CB_9"
  Generic_Relay_v2_8/1 -> Bus Creator6/8  "F2_CB_8"
  Generic_Relay_v2_7/1 -> Bus Creator6/7  "F2_CB_7"
  Generic_Relay_v2_2/1 -> Bus Creator6/2  "F2_CB_2"
  Generic_Relay_v2_3/1 -> Bus Creator6/3  "F2_CB_3"
  Generic_Relay_v2_4/1 -> Bus Creator6/4  "F2_CB_4"
  Generic_Relay_v2_5/1 -> Bus Creator6/5  "F2_CB_5"
  Generic_Relay_v2_6/1 -> Bus Creator6/6  "F2_CB_6"
  Generic_Relay_v2_17/1 -> Bus Creator6/17  "F2_CB_17"
  Bus Selector2/17 -> Generic_Relay_v2_17/1  "<F2_CB_17>"
  Modbus device18/1 -> Generic_Relay_v2_19/2
  Generic_Relay_v2_19/2 -> Modbus device18/1
  Modbus device17/1 -> Generic_Relay_v2_18/2
  Generic_Relay_v2_18/2 -> Modbus device17/1
  Generic_Relay_v2_18/1 -> Bus Creator6/18  "F2_CB_18"
  Generic_Relay_v2_19/1 -> Bus Creator6/19  "F2_CB_19"
  Bus Selector2/19 -> Generic_Relay_v2_19/1  "<F2_CB_19>"
  Bus Selector2/18 -> Generic_Relay_v2_18/1  "<F2_CB_18>"

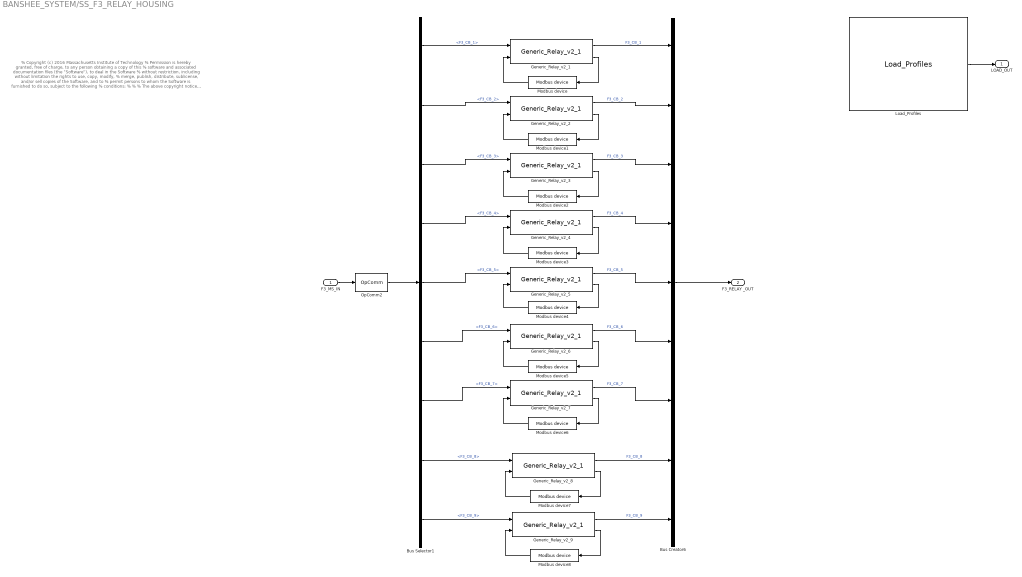
== system BANSHEE_SYSTEM/SS_F3_RELAY_HOUSING ==
  note: % Copyright (c) 2016 Massachusetts Institute of Technology
      | % Permission is hereby granted, free of charge, to any person obtaining a copy of this
      | % software and associated documentation files (the "Software"), to deal in the Software
      | % without restriction, including without limitation the rights to use, copy, modify,
      | % merge, publish, distribute, sublicense, and/or sell copies of the Software, and to
      | % permit persons to whom the Software is furnished to do so, subject to the following
      | % conditions:
      | %
      | %
      | % The above copyright notice and this permission notice shall be included in
      | % all copies or substantial portions of the Software.
      | %
      | % THE SOFTWARE IS PROVIDED "AS IS", WITHOUT WARRANTY OF ANY KIND, EXPRESS OR IMPLIED,
      | % INCLUDING BUT NOT LIMITED TO THE WARRANTIES OF MERCHANTABILITY, FITNESS FOR A
      | % PARTICULAR PURPOSE AND NONINFRINGEMENT. IN NO EVENT SHALL THE AUTHORS OR COPYRIGHT
      | % HOLDERS BE LIABLE FOR ANY CLAIM, DAMAGES OR OTHER LIABILITY, WHETHER IN AN ACTION
      | % OF CONTRACT, TORT OR OTHERWISE, ARISING FROM, OUT OF OR IN CONNECTION WITH THE
      | % SOFTWARE OR THE USE OR OTHER DEALINGS IN THE SOFTWARE.
      | %
      | %
      | %%
  F3_MS_IN : Inport
  Bus Creator6 : BusCreator  Inputs=9
  Bus Selector1 : BusSelector  OutputSignals=F3_CB_1,F3_CB_2,F3_CB_3,F3_CB_4,F3_CB_5,F3_CB_6,F3_CB_7,F3_CB_8,F3_CB_9
  Generic_Relay_v2_1 : relay_modbus_lib/Generic_Relay_v2_1  Ts=Ts  relay_settings=[F3(1,:)]
  Generic_Relay_v2_2 : relay_modbus_lib/Generic_Relay_v2_1  Ts=Ts  relay_settings=[F3(2,:)]
  Generic_Relay_v2_3 : relay_modbus_lib/Generic_Relay_v2_1  Ts=Ts  relay_settings=[F3(3,:)]
  Generic_Relay_v2_4 : relay_modbus_lib/Generic_Relay_v2_1  Ts=Ts  relay_settings=[F3(4,:)]
  Generic_Relay_v2_5 : relay_modbus_lib/Generic_Relay_v2_1  Ts=Ts  relay_settings=[F3(5,:)]
  Generic_Relay_v2_6 : relay_modbus_lib/Generic_Relay_v2_1  Ts=Ts  relay_settings=[F3(6,:)]
  Generic_Relay_v2_7 : relay_modbus_lib/Generic_Relay_v2_1  Ts=Ts  relay_settings=[F3(7,:)]
  Generic_Relay_v2_8 : relay_modbus_lib/Generic_Relay_v2_1  Ts=Ts  relay_settings=[F3(8,:)]
  Generic_Relay_v2_9 : relay_modbus_lib/Generic_Relay_v2_1  Ts=Ts  relay_settings=[F3(9,:)]
  Load_Profiles : LoadProfiles_lib/Load_Profiles
  Modbus device : rtio_generic_modbus/Modbus device  conf_name=F3_relay_cfg1.opal  conf_name_mask=F3_relay_cfg1.xls  sample_time=Ts
  Modbus device1 : rtio_generic_modbus/Modbus device  conf_name=F3_relay_cfg2.opal  conf_name_mask=F3_relay_cfg2.xls  sample_time=Ts
  Modbus device2 : rtio_generic_modbus/Modbus device  conf_name=F3_relay_cfg3.opal  conf_name_mask=F3_relay_cfg3.xls  sample_time=Ts
  Modbus device3 : rtio_generic_modbus/Modbus device  conf_name=F3_relay_cfg4.opal  conf_name_mask=F3_relay_cfg4.xls  sample_time=Ts
  Modbus device4 : rtio_generic_modbus/Modbus device  conf_name=F3_relay_cfg5.opal  conf_name_mask=F3_relay_cfg5.xls  sample_time=Ts
  Modbus device5 : rtio_generic_modbus/Modbus device  conf_name=F3_relay_cfg6.opal  conf_name_mask=F3_relay_cfg6.xls  sample_time=Ts
  Modbus device6 : rtio_generic_modbus/Modbus device  conf_name=F3_relay_cfg7.opal  conf_name_mask=F3_relay_cfg7.xls  sample_time=Ts
  Modbus device7 : rtio_generic_modbus/Modbus device  conf_name=F3_relay_cfg8.opal  conf_name_mask=F3_relay_cfg8.xls  sample_time=Ts
  Modbus device8 : rtio_generic_modbus/Modbus device  conf_name=F3_relay_cfg9.opal  conf_name_mask=F3_relay_cfg9.xls  sample_time=Ts
  OpComm2 : rtlab/OpComm  nbport=1  groupe_acq=1  subsys_rate=0  st=0  Synchronization=on  Interpolation=on  Threshold=1.0  Missed_Data=off  Sim_Time=off  Samples=off  dynSigOut=off  from_console=0  warning_done=off  writeOpCommFile=off  Offset=off
  LOAD_OUT : Outport
  F3_RELAY _OUT : Outport  Port=2
  wires:
  Load_Profiles/1 -> LOAD_OUT/1
  OpComm2/1 -> Bus Selector1/1
  Generic_Relay_v2_1/2 -> Modbus device/1
  Modbus device/1 -> Generic_Relay_v2_1/2
  Generic_Relay_v2_2/2 -> Modbus device1/1
  Modbus device1/1 -> Generic_Relay_v2_2/2
  Modbus device2/1 -> Generic_Relay_v2_3/2
  Generic_Relay_v2_3/2 -> Modbus device2/1
  Generic_Relay_v2_4/2 -> Modbus device3/1
  Modbus device3/1 -> Generic_Relay_v2_4/2
  Generic_Relay_v2_5/2 -> Modbus device4/1
  Modbus device4/1 -> Generic_Relay_v2_5/2
  Modbus device5/1 -> Generic_Relay_v2_6/2
  Generic_Relay_v2_6/2 -> Modbus device5/1
  Generic_Relay_v2_7/2 -> Modbus device6/1
  Modbus device6/1 -> Generic_Relay_v2_7/2
  F3_MS_IN/1 -> OpComm2/1
  Bus Selector1/1 -> Generic_Relay_v2_1/1  "<F3_CB_1>"
  Bus Selector1/2 -> Generic_Relay_v2_2/1  "<F3_CB_2>"
  Bus Selector1/3 -> Generic_Relay_v2_3/1  "<F3_CB_3>"
  Bus Selector1/4 -> Generic_Relay_v2_4/1  "<F3_CB_4>"
  Bus Selector1/5 -> Generic_Relay_v2_5/1  "<F3_CB_5>"
  Bus Selector1/6 -> Generic_Relay_v2_6/1  "<F3_CB_6>"
  Bus Selector1/7 -> Generic_Relay_v2_7/1  "<F3_CB_7>"
  Generic_Relay_v2_1/1 -> Bus Creator6/1  "F3_CB_1"
  Generic_Relay_v2_2/1 -> Bus Creator6/2  "F3_CB_2"
  Generic_Relay_v2_3/1 -> Bus Creator6/3  "F3_CB_3"
  Generic_Relay_v2_4/1 -> Bus Creator6/4  "F3_CB_4"
  Generic_Relay_v2_5/1 -> Bus Creator6/5  "F3_CB_5"
  Generic_Relay_v2_6/1 -> Bus Creator6/6  "F3_CB_6"
  Generic_Relay_v2_7/1 -> Bus Creator6/7  "F3_CB_7"
  Bus Creator6/1 -> F3_RELAY _OUT/1
  Modbus device7/1 -> Generic_Relay_v2_8/2
  Generic_Relay_v2_8/2 -> Modbus device7/1
  Generic_Relay_v2_9/2 -> Modbus device8/1
  Modbus device8/1 -> Generic_Relay_v2_9/2
  Generic_Relay_v2_8/1 -> Bus Creator6/8  "F3_CB_8"
  Generic_Relay_v2_9/1 -> Bus Creator6/9  "F3_CB_9"
  Bus Selector1/9 -> Generic_Relay_v2_9/1  "<F3_CB_9>"
  Bus Selector1/8 -> Generic_Relay_v2_8/1  "<F3_CB_8>"
